simulink model "T6_changeloadmodeltocurrentload_v1"  (R2022b)
settings: Solver=FixedStepAuto  StartTime=0.0  StopTime=48*4  FixedStep=0.01  RelTol=1e-3
undefined symbols (not defined in the file): cableLV, cableMV, High, Low, LV, MV, Scaling_factor, Ts
libraries: fl_lib x149, nesl_utility x73, simulink x60, ee_lib x9
(part 2 of 3)

== system T6_changeloadmodeltocurrentload_v1/Household2 ==
  note: I = P / U
  Constant : Constant  Value=LV
  Controlled Current Source : fl_lib/Electrical/Electrical Sources/Controlled Current Source
  Current Sensor : fl_lib/Electrical/Electrical Sensors/Current Sensor
  Divide : Product  Inputs=*/
  Gain : Gain  Gain=Scaling_factor
  MATLAB Function : MATLAB Function  TreatAsAtomicUnit=on
  PS-Simulink Converter : nesl_utility/PS-Simulink Converter  PhysicalDomain=network_engine_domain  SubClassName=ps_output  LeftPortType=input  RightPortType=output  PseudoPeriodic=off  Frequencies=[]  VectorFormat=inherit  Unit=inherit  AffineConversion=off
  PS-Simulink Converter1 : nesl_utility/PS-Simulink Converter  PhysicalDomain=network_engine_domain  SubClassName=ps_output  LeftPortType=input  RightPortType=output  PseudoPeriodic=off  Frequencies=[]  VectorFormat=inherit  Unit=inherit  AffineConversion=off
  Product : Product
  Repeating Sequence Interpolated : simulink/Sources/Repeating Sequence Interpolated  OutValues=Household15_Springallday  TimeValues=Allday_timevector  LookUpMeth=Interpolation-Use End Values  tsamp=0.01  OutMin=[]  OutMax=[]  OutDataTypeStr=double  OutputDataTypeScalingMode=double  OutDataType=fixdt(0,8)  OutScaling=2^-10
  Repeating Sequence Interpolated1 : simulink/Sources/Repeating Sequence Interpolated  OutValues=Household15_Summerallday  TimeValues=Allday_timevector  LookUpMeth=Interpolation-Use End Values  tsamp=0.01  OutMin=[]  OutMax=[]  OutDataTypeStr=double  OutputDataTypeScalingMode=double  OutDataType=fixdt(0,8)  OutScaling=2^-10
  Repeating Sequence Interpolated2 : simulink/Sources/Repeating Sequence Interpolated  OutValues=Household15_Autumnallday  TimeValues=Allday_timevector  LookUpMeth=Interpolation-Use End Values  tsamp=0.01  OutMin=[]  OutMax=[]  OutDataTypeStr=double  OutputDataTypeScalingMode=double  OutDataType=fixdt(0,8)  OutScaling=2^-10
  Repeating Sequence Interpolated3 : simulink/Sources/Repeating Sequence Interpolated  OutValues=Household15_Winterallday  TimeValues=Allday_timevector  LookUpMeth=Interpolation-Use End Values  tsamp=0.01  OutMin=[]  OutMax=[]  OutDataTypeStr=double  OutputDataTypeScalingMode=double  OutDataType=fixdt(0,8)  OutScaling=2^-10
  Scope : Scope
  Simscape Bus1 : SimscapeBus  HierarchyStrings=High;Low
  Simulink-PS Converter1 : nesl_utility/Simulink-PS Converter  PhysicalDomain=network_engine_domain  SubClassName=ps_input  LeftPortType=input  RightPortType=output  PseudoPeriodic=off  Frequencies=[]  NoiseDistribution=none  NoiseParameters=[]  Unit=A  AffineConversion=off  FilteringAndDerivatives=provide  SimscapeFilterOrder=1  InputFilterTimeConstant=0.001  UdotUserProvided=0
  Voltage Sensor : fl_lib/Electrical/Electrical Sensors/Voltage Sensor
  IndustrialOut : PMIOPort  Side=Right
  tag scope: Residential_power2=global
  wires:
  Repeating Sequence Interpolated3/1 -> MATLAB Function/8(data4)
  Repeating Sequence Interpolated2/1 -> MATLAB Function/7(data3)
  Repeating Sequence Interpolated1/1 -> MATLAB Function/6(data2)
  Repeating Sequence Interpolated/1 -> MATLAB Function/5(data1)
  [Button1selected] -> MATLAB Function/1(button1)
  [Button2selected] -> MATLAB Function/2(button2)
  [Button3selected] -> MATLAB Function/3(button3)
  [Button4selected] -> MATLAB Function/4(button4)
  Product/1 -> [Residential_power2]  "power"
  PS-Simulink Converter1/1 -> Product/1  "current"
  PS-Simulink Converter/1 -> Product/2  "voltage"
  MATLAB Function/1(y) -> Gain/1, Scope/1  "electrical"
  Divide/1 -> Simulink-PS Converter1/1
  Gain/1 -> Divide/1
  Constant/1 -> Divide/2
  connections:
  Current Sensor/LConn1 -- Simscape Bus1/LConn1
  Current Sensor/RConn1 -- PS-Simulink Converter1/LConn1
  Voltage Sensor/RConn1 -- PS-Simulink Converter/LConn1
  Current Sensor/RConn2 -- Controlled Current Source/RConn2 -- Voltage Sensor/LConn1
  IndustrialOut/RConn1 -- Simscape Bus1/RConn1
  Voltage Sensor/RConn2 -- Simscape Bus1/LConn2 -- Controlled Current Source/LConn1
  Simulink-PS Converter1/RConn1 -- Controlled Current Source/RConn1

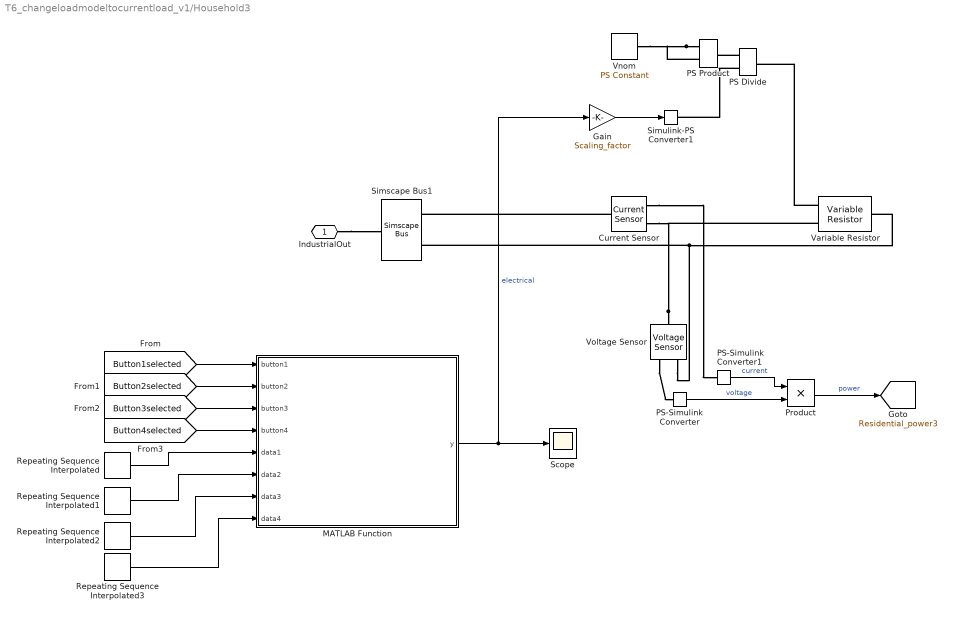
== system T6_changeloadmodeltocurrentload_v1/Household3 ==
  Current Sensor : fl_lib/Electrical/Electrical Sensors/Current Sensor
  Gain : Gain  Gain=Scaling_factor
  MATLAB Function : MATLAB Function  TreatAsAtomicUnit=on
  PS Divide : fl_lib/Physical Signals/Functions/PS Divide
  PS Product : fl_lib/Physical Signals/Functions/PS Product
  PS-Simulink Converter : nesl_utility/PS-Simulink Converter  PhysicalDomain=network_engine_domain  SubClassName=ps_output  LeftPortType=input  RightPortType=output  PseudoPeriodic=off  Frequencies=[]  VectorFormat=inherit  Unit=inherit  AffineConversion=off
  PS-Simulink Converter1 : nesl_utility/PS-Simulink Converter  PhysicalDomain=network_engine_domain  SubClassName=ps_output  LeftPortType=input  RightPortType=output  PseudoPeriodic=off  Frequencies=[]  VectorFormat=inherit  Unit=inherit  AffineConversion=off
  Product : Product
  Repeating Sequence Interpolated : simulink/Sources/Repeating Sequence Interpolated  OutValues=Household8_Springallday  TimeValues=Allday_timevector  LookUpMeth=Interpolation-Use End Values  tsamp=0.01  OutMin=[]  OutMax=[]  OutDataTypeStr=double  OutputDataTypeScalingMode=double  OutDataType=fixdt(0,8)  OutScaling=2^-10
  Repeating Sequence Interpolated1 : simulink/Sources/Repeating Sequence Interpolated  OutValues=Household8_Summerallday  TimeValues=Allday_timevector  LookUpMeth=Interpolation-Use End Values  tsamp=0.01  OutMin=[]  OutMax=[]  OutDataTypeStr=double  OutputDataTypeScalingMode=double  OutDataType=fixdt(0,8)  OutScaling=2^-10
  Repeating Sequence Interpolated2 : simulink/Sources/Repeating Sequence Interpolated  OutValues=Household8_Autumnallday  TimeValues=Allday_timevector  LookUpMeth=Interpolation-Use End Values  tsamp=0.01  OutMin=[]  OutMax=[]  OutDataTypeStr=double  OutputDataTypeScalingMode=double  OutDataType=fixdt(0,8)  OutScaling=2^-10
  Repeating Sequence Interpolated3 : simulink/Sources/Repeating Sequence Interpolated  OutValues=Household8_Winterallday  TimeValues=Allday_timevector  LookUpMeth=Interpolation-Use End Values  tsamp=0.01  OutMin=[]  OutMax=[]  OutDataTypeStr=double  OutputDataTypeScalingMode=double  OutDataType=fixdt(0,8)  OutScaling=2^-10
  Scope : Scope
  Simscape Bus1 : SimscapeBus  HierarchyStrings=High;Low
  Simulink-PS Converter1 : nesl_utility/Simulink-PS Converter  PhysicalDomain=network_engine_domain  SubClassName=ps_input  LeftPortType=input  RightPortType=output  PseudoPeriodic=off  Frequencies=[]  NoiseDistribution=none  NoiseParameters=[]  Unit=V*A  AffineConversion=off  FilteringAndDerivatives=provide  SimscapeFilterOrder=1  InputFilterTimeConstant=0.001  UdotUserProvided=0
  Variable Resistor : fl_lib/Electrical/Electrical Elements/Variable Resistor  Rmin=0 Ohm  i_specify=off  i_priority=None  i=0 A  i_nominal_specify=off  i_nominal_unit=A  i_nominal_value=1  v_specify=off  v_priority=None  v=0 V  v_nominal_specify=off  v_nominal_unit=V  v_nominal_value=1
  Vnom : fl_lib/Physical Signals/Sources/PS Constant  constant=LV V
  Voltage Sensor : fl_lib/Electrical/Electrical Sensors/Voltage Sensor
  IndustrialOut : PMIOPort  Side=Right
  tag scope: Residential_power3=global
  wires:
  MATLAB Function/1(y) -> Gain/1, Scope/1  "electrical"
  PS-Simulink Converter/1 -> Product/2  "voltage"
  PS-Simulink Converter1/1 -> Product/1  "current"
  Product/1 -> [Residential_power3]  "power"
  [Button4selected] -> MATLAB Function/4(button4)
  [Button3selected] -> MATLAB Function/3(button3)
  [Button2selected] -> MATLAB Function/2(button2)
  [Button1selected] -> MATLAB Function/1(button1)
  Repeating Sequence Interpolated/1 -> MATLAB Function/5(data1)
  Repeating Sequence Interpolated1/1 -> MATLAB Function/6(data2)
  Repeating Sequence Interpolated2/1 -> MATLAB Function/7(data3)
  Repeating Sequence Interpolated3/1 -> MATLAB Function/8(data4)
  Gain/1 -> Simulink-PS Converter1/1
  connections:
  PS Divide/LConn1 -- PS Product/RConn1
  Variable Resistor/LConn1 -- PS Divide/RConn1
  PS Divide/LConn2 -- Simulink-PS Converter1/RConn1
  PS Product/LConn1 -- PS Product/LConn2 -- Vnom/RConn1
  Voltage Sensor/RConn2 -- Simscape Bus1/LConn2 -- Variable Resistor/RConn1
  IndustrialOut/RConn1 -- Simscape Bus1/RConn1
  Voltage Sensor/LConn1 -- Variable Resistor/LConn2 -- Current Sensor/RConn2
  Voltage Sensor/RConn1 -- PS-Simulink Converter/LConn1
  Current Sensor/RConn1 -- PS-Simulink Converter1/LConn1
  Current Sensor/LConn1 -- Simscape Bus1/LConn1

== system T6_changeloadmodeltocurrentload_v1/Household4 ==
  Current Sensor : fl_lib/Electrical/Electrical Sensors/Current Sensor
  Gain : Gain  Gain=Scaling_factor
  MATLAB Function : MATLAB Function  TreatAsAtomicUnit=on
  PS Divide : fl_lib/Physical Signals/Functions/PS Divide
  PS Product : fl_lib/Physical Signals/Functions/PS Product
  PS-Simulink Converter : nesl_utility/PS-Simulink Converter  PhysicalDomain=network_engine_domain  SubClassName=ps_output  LeftPortType=input  RightPortType=output  PseudoPeriodic=off  Frequencies=[]  VectorFormat=inherit  Unit=inherit  AffineConversion=off
  PS-Simulink Converter1 : nesl_utility/PS-Simulink Converter  PhysicalDomain=network_engine_domain  SubClassName=ps_output  LeftPortType=input  RightPortType=output  PseudoPeriodic=off  Frequencies=[]  VectorFormat=inherit  Unit=inherit  AffineConversion=off
  Product : Product
  Repeating Sequence Interpolated : simulink/Sources/Repeating Sequence Interpolated  OutValues=Household4_Springallday  TimeValues=Allday_timevector  LookUpMeth=Interpolation-Use End Values  tsamp=0.01  OutMin=[]  OutMax=[]  OutDataTypeStr=double  OutputDataTypeScalingMode=double  OutDataType=fixdt(0,8)  OutScaling=2^-10
  Repeating Sequence Interpolated1 : simulink/Sources/Repeating Sequence Interpolated  OutValues=Household4_Summerallday  TimeValues=Allday_timevector  LookUpMeth=Interpolation-Use End Values  tsamp=0.01  OutMin=[]  OutMax=[]  OutDataTypeStr=double  OutputDataTypeScalingMode=double  OutDataType=fixdt(0,8)  OutScaling=2^-10
  Repeating Sequence Interpolated2 : simulink/Sources/Repeating Sequence Interpolated  OutValues=Household4_Autumnallday  TimeValues=Allday_timevector  LookUpMeth=Interpolation-Use End Values  tsamp=0.01  OutMin=[]  OutMax=[]  OutDataTypeStr=double  OutputDataTypeScalingMode=double  OutDataType=fixdt(0,8)  OutScaling=2^-10
  Repeating Sequence Interpolated3 : simulink/Sources/Repeating Sequence Interpolated  OutValues=Household4_Winterallday  TimeValues=Allday_timevector  LookUpMeth=Interpolation-Use End Values  tsamp=0.01  OutMin=[]  OutMax=[]  OutDataTypeStr=double  OutputDataTypeScalingMode=double  OutDataType=fixdt(0,8)  OutScaling=2^-10
  Scope : Scope
  Simscape Bus1 : SimscapeBus  HierarchyStrings=High;Low
  Simulink-PS Converter1 : nesl_utility/Simulink-PS Converter  PhysicalDomain=network_engine_domain  SubClassName=ps_input  LeftPortType=input  RightPortType=output  PseudoPeriodic=off  Frequencies=[]  NoiseDistribution=none  NoiseParameters=[]  Unit=V*A  AffineConversion=off  FilteringAndDerivatives=provide  SimscapeFilterOrder=1  InputFilterTimeConstant=0.001  UdotUserProvided=0
  Variable Resistor : fl_lib/Electrical/Electrical Elements/Variable Resistor  Rmin=0 Ohm  i_specify=off  i_priority=None  i=0 A  i_nominal_specify=off  i_nominal_unit=A  i_nominal_value=1  v_specify=off  v_priority=None  v=0 V  v_nominal_specify=off  v_nominal_unit=V  v_nominal_value=1
  Vnom : fl_lib/Physical Signals/Sources/PS Constant  constant=LV V
  Voltage Sensor : fl_lib/Electrical/Electrical Sensors/Voltage Sensor
  IndustrialOut : PMIOPort  Side=Right
  tag scope: Residential_power4=global
  wires:
  Repeating Sequence Interpolated3/1 -> MATLAB Function/8(data4)
  Repeating Sequence Interpolated2/1 -> MATLAB Function/7(data3)
  Repeating Sequence Interpolated1/1 -> MATLAB Function/6(data2)
  Repeating Sequence Interpolated/1 -> MATLAB Function/5(data1)
  [Button1selected] -> MATLAB Function/1(button1)
  [Button2selected] -> MATLAB Function/2(button2)
  [Button3selected] -> MATLAB Function/3(button3)
  [Button4selected] -> MATLAB Function/4(button4)
  Product/1 -> [Residential_power4]  "power"
  PS-Simulink Converter1/1 -> Product/1  "current"
  PS-Simulink Converter/1 -> Product/2  "voltage"
  MATLAB Function/1(y) -> Gain/1, Scope/1  "electrical"
  Gain/1 -> Simulink-PS Converter1/1
  connections:
  Current Sensor/LConn1 -- Simscape Bus1/LConn1
  Current Sensor/RConn1 -- PS-Simulink Converter1/LConn1
  Voltage Sensor/RConn1 -- PS-Simulink Converter/LConn1
  Current Sensor/RConn2 -- Variable Resistor/LConn2 -- Voltage Sensor/LConn1
  IndustrialOut/RConn1 -- Simscape Bus1/RConn1
  Variable Resistor/RConn1 -- Simscape Bus1/LConn2 -- Voltage Sensor/RConn2
  Vnom/RConn1 -- PS Product/LConn2 -- PS Product/LConn1
  PS Divide/LConn2 -- Simulink-PS Converter1/RConn1
  Variable Resistor/LConn1 -- PS Divide/RConn1
  PS Divide/LConn1 -- PS Product/RConn1

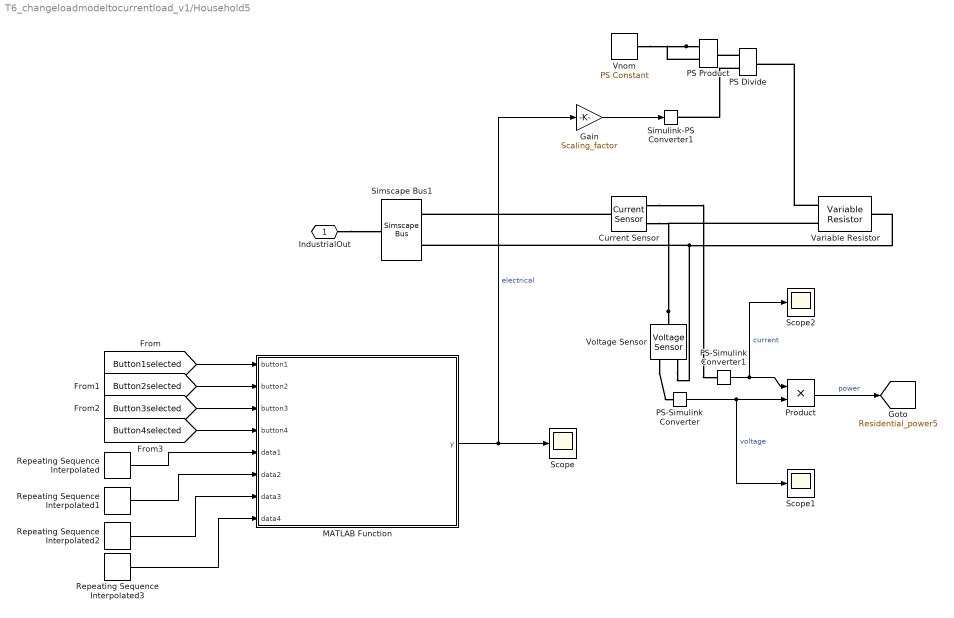
== system T6_changeloadmodeltocurrentload_v1/Household5 ==
  Current Sensor : fl_lib/Electrical/Electrical Sensors/Current Sensor
  Gain : Gain  Gain=Scaling_factor
  MATLAB Function : MATLAB Function  TreatAsAtomicUnit=on
  PS Divide : fl_lib/Physical Signals/Functions/PS Divide
  PS Product : fl_lib/Physical Signals/Functions/PS Product
  PS-Simulink Converter : nesl_utility/PS-Simulink Converter  PhysicalDomain=network_engine_domain  SubClassName=ps_output  LeftPortType=input  RightPortType=output  PseudoPeriodic=off  Frequencies=[]  VectorFormat=inherit  Unit=inherit  AffineConversion=off
  PS-Simulink Converter1 : nesl_utility/PS-Simulink Converter  PhysicalDomain=network_engine_domain  SubClassName=ps_output  LeftPortType=input  RightPortType=output  PseudoPeriodic=off  Frequencies=[]  VectorFormat=inherit  Unit=inherit  AffineConversion=off
  Product : Product
  Repeating Sequence Interpolated : simulink/Sources/Repeating Sequence Interpolated  OutValues=Household26_Springallday  TimeValues=Allday_timevector  LookUpMeth=Interpolation-Use End Values  tsamp=0.01  OutMin=[]  OutMax=[]  OutDataTypeStr=double  OutputDataTypeScalingMode=double  OutDataType=fixdt(0,8)  OutScaling=2^-10
  Repeating Sequence Interpolated1 : simulink/Sources/Repeating Sequence Interpolated  OutValues=Household26_Summerallday  TimeValues=Allday_timevector  LookUpMeth=Interpolation-Use End Values  tsamp=0.01  OutMin=[]  OutMax=[]  OutDataTypeStr=double  OutputDataTypeScalingMode=double  OutDataType=fixdt(0,8)  OutScaling=2^-10
  Repeating Sequence Interpolated2 : simulink/Sources/Repeating Sequence Interpolated  OutValues=Household26_Autumnallday  TimeValues=Allday_timevector  LookUpMeth=Interpolation-Use End Values  tsamp=0.01  OutMin=[]  OutMax=[]  OutDataTypeStr=double  OutputDataTypeScalingMode=double  OutDataType=fixdt(0,8)  OutScaling=2^-10
  Repeating Sequence Interpolated3 : simulink/Sources/Repeating Sequence Interpolated  OutValues=Household26_Winterallday  TimeValues=Allday_timevector  LookUpMeth=Interpolation-Use End Values  tsamp=0.01  OutMin=[]  OutMax=[]  OutDataTypeStr=double  OutputDataTypeScalingMode=double  OutDataType=fixdt(0,8)  OutScaling=2^-10
  Scope : Scope
  Scope1 : Scope
  Scope2 : Scope
  Simscape Bus1 : SimscapeBus  HierarchyStrings=High;Low
  Simulink-PS Converter1 : nesl_utility/Simulink-PS Converter  PhysicalDomain=network_engine_domain  SubClassName=ps_input  LeftPortType=input  RightPortType=output  PseudoPeriodic=off  Frequencies=[]  NoiseDistribution=none  NoiseParameters=[]  Unit=V*A  AffineConversion=off  FilteringAndDerivatives=provide  SimscapeFilterOrder=1  InputFilterTimeConstant=0.001  UdotUserProvided=0
  Variable Resistor : fl_lib/Electrical/Electrical Elements/Variable Resistor  Rmin=0 Ohm  i_specify=off  i_priority=None  i=0 A  i_nominal_specify=off  i_nominal_unit=A  i_nominal_value=1  v_specify=off  v_priority=None  v=0 V  v_nominal_specify=off  v_nominal_unit=V  v_nominal_value=1
  Vnom : fl_lib/Physical Signals/Sources/PS Constant  constant=LV V
  Voltage Sensor : fl_lib/Electrical/Electrical Sensors/Voltage Sensor
  IndustrialOut : PMIOPort  Side=Right
  tag scope: Residential_power5=global
  wires:
  MATLAB Function/1(y) -> Gain/1, Scope/1  "electrical"
  PS-Simulink Converter/1 -> Scope1/1, Product/2  "voltage"
  PS-Simulink Converter1/1 -> Scope2/1, Product/1  "current"
  Product/1 -> [Residential_power5]  "power"
  [Button4selected] -> MATLAB Function/4(button4)
  [Button3selected] -> MATLAB Function/3(button3)
  [Button2selected] -> MATLAB Function/2(button2)
  [Button1selected] -> MATLAB Function/1(button1)
  Repeating Sequence Interpolated/1 -> MATLAB Function/5(data1)
  Repeating Sequence Interpolated1/1 -> MATLAB Function/6(data2)
  Repeating Sequence Interpolated2/1 -> MATLAB Function/7(data3)
  Repeating Sequence Interpolated3/1 -> MATLAB Function/8(data4)
  Gain/1 -> Simulink-PS Converter1/1
  connections:
  PS Divide/LConn1 -- PS Product/RConn1
  Variable Resistor/LConn1 -- PS Divide/RConn1
  PS Divide/LConn2 -- Simulink-PS Converter1/RConn1
  PS Product/LConn1 -- PS Product/LConn2 -- Vnom/RConn1
  Voltage Sensor/RConn2 -- Simscape Bus1/LConn2 -- Variable Resistor/RConn1
  IndustrialOut/RConn1 -- Simscape Bus1/RConn1
  Voltage Sensor/LConn1 -- Variable Resistor/LConn2 -- Current Sensor/RConn2
  Voltage Sensor/RConn1 -- PS-Simulink Converter/LConn1
  Current Sensor/RConn1 -- PS-Simulink Converter1/LConn1
  Current Sensor/LConn1 -- Simscape Bus1/LConn1

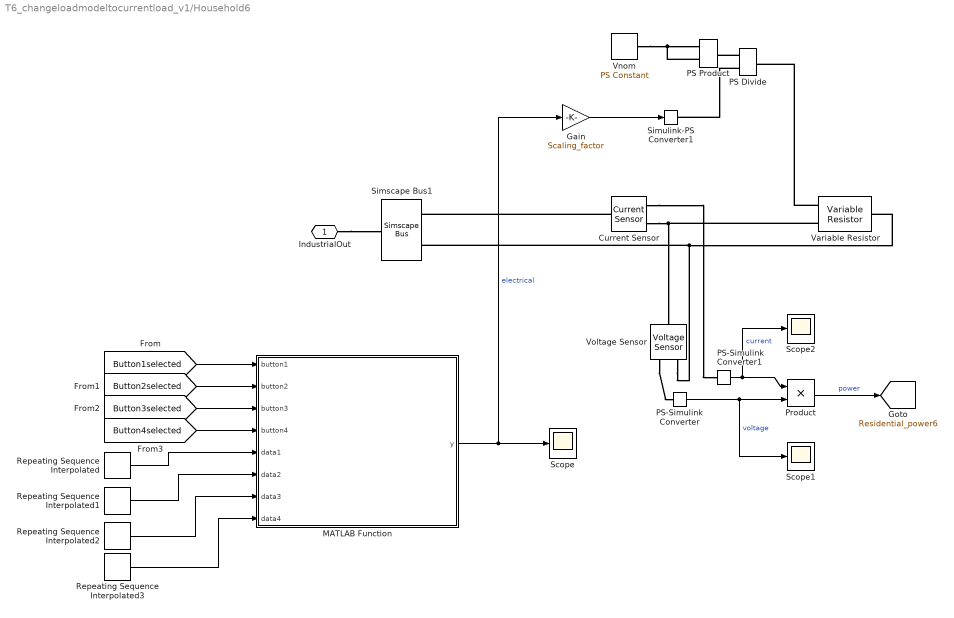
== system T6_changeloadmodeltocurrentload_v1/Household6 ==
  Current Sensor : fl_lib/Electrical/Electrical Sensors/Current Sensor
  Gain : Gain  Gain=Scaling_factor
  MATLAB Function : MATLAB Function  TreatAsAtomicUnit=on
  PS Divide : fl_lib/Physical Signals/Functions/PS Divide
  PS Product : fl_lib/Physical Signals/Functions/PS Product
  PS-Simulink Converter : nesl_utility/PS-Simulink Converter  PhysicalDomain=network_engine_domain  SubClassName=ps_output  LeftPortType=input  RightPortType=output  PseudoPeriodic=off  Frequencies=[]  VectorFormat=inherit  Unit=inherit  AffineConversion=off
  PS-Simulink Converter1 : nesl_utility/PS-Simulink Converter  PhysicalDomain=network_engine_domain  SubClassName=ps_output  LeftPortType=input  RightPortType=output  PseudoPeriodic=off  Frequencies=[]  VectorFormat=inherit  Unit=inherit  AffineConversion=off
  Product : Product
  Repeating Sequence Interpolated : simulink/Sources/Repeating Sequence Interpolated  OutValues=Household9_Springallday  TimeValues=Allday_timevector  LookUpMeth=Interpolation-Use End Values  tsamp=0.01  OutMin=[]  OutMax=[]  OutDataTypeStr=double  OutputDataTypeScalingMode=double  OutDataType=fixdt(0,8)  OutScaling=2^-10
  Repeating Sequence Interpolated1 : simulink/Sources/Repeating Sequence Interpolated  OutValues=Household9_Summerallday  TimeValues=Allday_timevector  LookUpMeth=Interpolation-Use End Values  tsamp=0.01  OutMin=[]  OutMax=[]  OutDataTypeStr=double  OutputDataTypeScalingMode=double  OutDataType=fixdt(0,8)  OutScaling=2^-10
  Repeating Sequence Interpolated2 : simulink/Sources/Repeating Sequence Interpolated  OutValues=Household9_Autumnallday  TimeValues=Allday_timevector  LookUpMeth=Interpolation-Use End Values  tsamp=0.01  OutMin=[]  OutMax=[]  OutDataTypeStr=double  OutputDataTypeScalingMode=double  OutDataType=fixdt(0,8)  OutScaling=2^-10
  Repeating Sequence Interpolated3 : simulink/Sources/Repeating Sequence Interpolated  OutValues=Household9_Winterallday  TimeValues=Allday_timevector  LookUpMeth=Interpolation-Use End Values  tsamp=0.01  OutMin=[]  OutMax=[]  OutDataTypeStr=double  OutputDataTypeScalingMode=double  OutDataType=fixdt(0,8)  OutScaling=2^-10
  Scope : Scope
  Scope1 : Scope
  Scope2 : Scope
  Simscape Bus1 : SimscapeBus  HierarchyStrings=High;Low
  Simulink-PS Converter1 : nesl_utility/Simulink-PS Converter  PhysicalDomain=network_engine_domain  SubClassName=ps_input  LeftPortType=input  RightPortType=output  PseudoPeriodic=off  Frequencies=[]  NoiseDistribution=none  NoiseParameters=[]  Unit=V*A  AffineConversion=off  FilteringAndDerivatives=provide  SimscapeFilterOrder=1  InputFilterTimeConstant=0.001  UdotUserProvided=0
  Variable Resistor : fl_lib/Electrical/Electrical Elements/Variable Resistor  Rmin=0 Ohm  i_specify=off  i_priority=None  i=0 A  i_nominal_specify=off  i_nominal_unit=A  i_nominal_value=1  v_specify=off  v_priority=None  v=0 V  v_nominal_specify=off  v_nominal_unit=V  v_nominal_value=1
  Vnom : fl_lib/Physical Signals/Sources/PS Constant  constant=LV V
  Voltage Sensor : fl_lib/Electrical/Electrical Sensors/Voltage Sensor
  IndustrialOut : PMIOPort  Side=Right
  tag scope: Residential_power6=global
  wires:
  Repeating Sequence Interpolated3/1 -> MATLAB Function/8(data4)
  Repeating Sequence Interpolated2/1 -> MATLAB Function/7(data3)
  Repeating Sequence Interpolated1/1 -> MATLAB Function/6(data2)
  Repeating Sequence Interpolated/1 -> MATLAB Function/5(data1)
  [Button1selected] -> MATLAB Function/1(button1)
  [Button2selected] -> MATLAB Function/2(button2)
  [Button3selected] -> MATLAB Function/3(button3)
  [Button4selected] -> MATLAB Function/4(button4)
  Product/1 -> [Residential_power6]  "power"
  PS-Simulink Converter1/1 -> Scope2/1, Product/1  "current"
  PS-Simulink Converter/1 -> Scope1/1, Product/2  "voltage"
  MATLAB Function/1(y) -> Gain/1, Scope/1  "electrical"
  Gain/1 -> Simulink-PS Converter1/1
  connections:
  Current Sensor/LConn1 -- Simscape Bus1/LConn1
  Current Sensor/RConn1 -- PS-Simulink Converter1/LConn1
  Voltage Sensor/RConn1 -- PS-Simulink Converter/LConn1
  Current Sensor/RConn2 -- Variable Resistor/LConn2 -- Voltage Sensor/LConn1
  IndustrialOut/RConn1 -- Simscape Bus1/RConn1
  Variable Resistor/RConn1 -- Simscape Bus1/LConn2 -- Voltage Sensor/RConn2
  Vnom/RConn1 -- PS Product/LConn2 -- PS Product/LConn1
  PS Divide/LConn2 -- Simulink-PS Converter1/RConn1
  Variable Resistor/LConn1 -- PS Divide/RConn1
  PS Divide/LConn1 -- PS Product/RConn1

== system T6_changeloadmodeltocurrentload_v1/Household7 ==
  Current Sensor : fl_lib/Electrical/Electrical Sensors/Current Sensor
  Gain : Gain  Gain=Scaling_factor
  MATLAB Function : MATLAB Function  TreatAsAtomicUnit=on
  PS Divide : fl_lib/Physical Signals/Functions/PS Divide
  PS Product : fl_lib/Physical Signals/Functions/PS Product
  PS-Simulink Converter : nesl_utility/PS-Simulink Converter  PhysicalDomain=network_engine_domain  SubClassName=ps_output  LeftPortType=input  RightPortType=output  PseudoPeriodic=off  Frequencies=[]  VectorFormat=inherit  Unit=inherit  AffineConversion=off
  PS-Simulink Converter1 : nesl_utility/PS-Simulink Converter  PhysicalDomain=network_engine_domain  SubClassName=ps_output  LeftPortType=input  RightPortType=output  PseudoPeriodic=off  Frequencies=[]  VectorFormat=inherit  Unit=inherit  AffineConversion=off
  Product : Product
  Repeating Sequence Interpolated : simulink/Sources/Repeating Sequence Interpolated  OutValues=Household5_Springallday  TimeValues=Allday_timevector  LookUpMeth=Interpolation-Use End Values  tsamp=0.01  OutMin=[]  OutMax=[]  OutDataTypeStr=double  OutputDataTypeScalingMode=double  OutDataType=fixdt(0,8)  OutScaling=2^-10
  Repeating Sequence Interpolated1 : simulink/Sources/Repeating Sequence Interpolated  OutValues=Household5_Summerallday  TimeValues=Allday_timevector  LookUpMeth=Interpolation-Use End Values  tsamp=0.01  OutMin=[]  OutMax=[]  OutDataTypeStr=double  OutputDataTypeScalingMode=double  OutDataType=fixdt(0,8)  OutScaling=2^-10
  Repeating Sequence Interpolated2 : simulink/Sources/Repeating Sequence Interpolated  OutValues=Household5_Autumnallday  TimeValues=Allday_timevector  LookUpMeth=Interpolation-Use End Values  tsamp=0.01  OutMin=[]  OutMax=[]  OutDataTypeStr=double  OutputDataTypeScalingMode=double  OutDataType=fixdt(0,8)  OutScaling=2^-10
  Repeating Sequence Interpolated3 : simulink/Sources/Repeating Sequence Interpolated  OutValues=Household5_Winterallday  TimeValues=Allday_timevector  LookUpMeth=Interpolation-Use End Values  tsamp=0.01  OutMin=[]  OutMax=[]  OutDataTypeStr=double  OutputDataTypeScalingMode=double  OutDataType=fixdt(0,8)  OutScaling=2^-10
  Scope : Scope
  Simscape Bus1 : SimscapeBus  HierarchyStrings=High;Low
  Simulink-PS Converter1 : nesl_utility/Simulink-PS Converter  PhysicalDomain=network_engine_domain  SubClassName=ps_input  LeftPortType=input  RightPortType=output  PseudoPeriodic=off  Frequencies=[]  NoiseDistribution=none  NoiseParameters=[]  Unit=V*A  AffineConversion=off  FilteringAndDerivatives=provide  SimscapeFilterOrder=1  InputFilterTimeConstant=0.001  UdotUserProvided=0
  Variable Resistor : fl_lib/Electrical/Electrical Elements/Variable Resistor  Rmin=0 Ohm  i_specify=off  i_priority=None  i=0 A  i_nominal_specify=off  i_nominal_unit=A  i_nominal_value=1  v_specify=off  v_priority=None  v=0 V  v_nominal_specify=off  v_nominal_unit=V  v_nominal_value=1
  Vnom : fl_lib/Physical Signals/Sources/PS Constant  constant=LV V
  Voltage Sensor : fl_lib/Electrical/Electrical Sensors/Voltage Sensor
  IndustrialOut : PMIOPort  Side=Right
  tag scope: Residential_power7=global
  wires:
  MATLAB Function/1(y) -> Gain/1, Scope/1  "electrical"
  PS-Simulink Converter/1 -> Product/2  "voltage"
  PS-Simulink Converter1/1 -> Product/1  "current"
  Product/1 -> [Residential_power7]  "power"
  [Button4selected] -> MATLAB Function/4(button4)
  [Button3selected] -> MATLAB Function/3(button3)
  [Button2selected] -> MATLAB Function/2(button2)
  [Button1selected] -> MATLAB Function/1(button1)
  Repeating Sequence Interpolated/1 -> MATLAB Function/5(data1)
  Repeating Sequence Interpolated1/1 -> MATLAB Function/6(data2)
  Repeating Sequence Interpolated2/1 -> MATLAB Function/7(data3)
  Repeating Sequence Interpolated3/1 -> MATLAB Function/8(data4)
  Gain/1 -> Simulink-PS Converter1/1
  connections:
  PS Divide/LConn1 -- PS Product/RConn1
  Variable Resistor/LConn1 -- PS Divide/RConn1
  PS Divide/LConn2 -- Simulink-PS Converter1/RConn1
  PS Product/LConn1 -- PS Product/LConn2 -- Vnom/RConn1
  Voltage Sensor/RConn2 -- Simscape Bus1/LConn2 -- Variable Resistor/RConn1
  IndustrialOut/RConn1 -- Simscape Bus1/RConn1
  Voltage Sensor/LConn1 -- Variable Resistor/LConn2 -- Current Sensor/RConn2
  Voltage Sensor/RConn1 -- PS-Simulink Converter/LConn1
  Current Sensor/RConn1 -- PS-Simulink Converter1/LConn1
  Current Sensor/LConn1 -- Simscape Bus1/LConn1

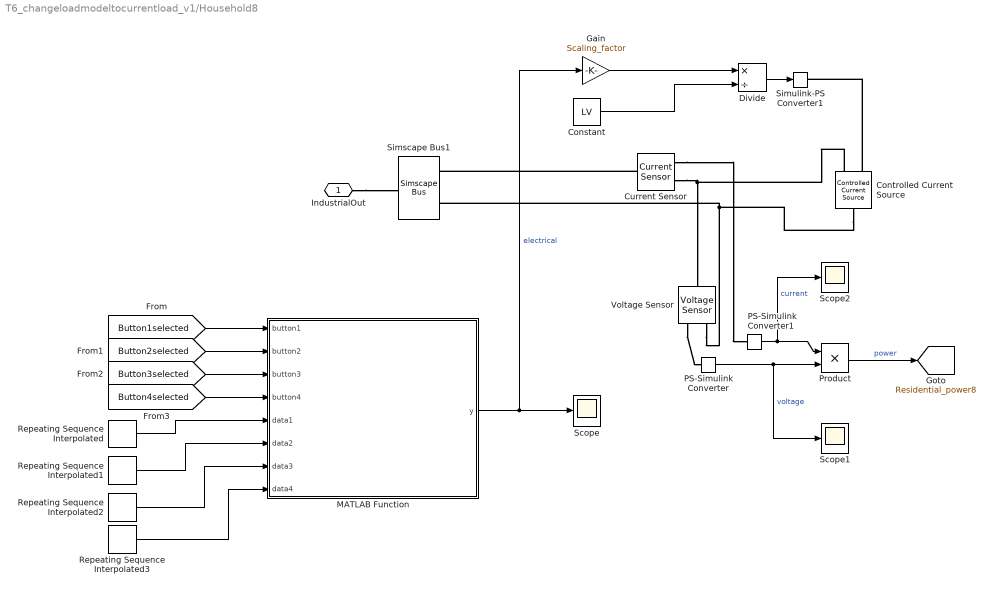
== system T6_changeloadmodeltocurrentload_v1/Household8 ==
  Constant : Constant  Value=LV
  Controlled Current Source : fl_lib/Electrical/Electrical Sources/Controlled Current Source
  Current Sensor : fl_lib/Electrical/Electrical Sensors/Current Sensor
  Divide : Product  Inputs=*/
  Gain : Gain  Gain=Scaling_factor
  MATLAB Function : MATLAB Function  TreatAsAtomicUnit=on
  PS-Simulink Converter : nesl_utility/PS-Simulink Converter  PhysicalDomain=network_engine_domain  SubClassName=ps_output  LeftPortType=input  RightPortType=output  PseudoPeriodic=off  Frequencies=[]  VectorFormat=inherit  Unit=inherit  AffineConversion=off
  PS-Simulink Converter1 : nesl_utility/PS-Simulink Converter  PhysicalDomain=network_engine_domain  SubClassName=ps_output  LeftPortType=input  RightPortType=output  PseudoPeriodic=off  Frequencies=[]  VectorFormat=inherit  Unit=inherit  AffineConversion=off
  Product : Product
  Repeating Sequence Interpolated : simulink/Sources/Repeating Sequence Interpolated  OutValues=Household33_Springallday  TimeValues=Allday_timevector  LookUpMeth=Interpolation-Use End Values  tsamp=0.01  OutMin=[]  OutMax=[]  OutDataTypeStr=double  OutputDataTypeScalingMode=double  OutDataType=fixdt(0,8)  OutScaling=2^-10
  Repeating Sequence Interpolated1 : simulink/Sources/Repeating Sequence Interpolated  OutValues=Household33_Summerallday  TimeValues=Allday_timevector  LookUpMeth=Interpolation-Use End Values  tsamp=0.01  OutMin=[]  OutMax=[]  OutDataTypeStr=double  OutputDataTypeScalingMode=double  OutDataType=fixdt(0,8)  OutScaling=2^-10
  Repeating Sequence Interpolated2 : simulink/Sources/Repeating Sequence Interpolated  OutValues=Household33_Autumnallday  TimeValues=Allday_timevector  LookUpMeth=Interpolation-Use End Values  tsamp=0.01  OutMin=[]  OutMax=[]  OutDataTypeStr=double  OutputDataTypeScalingMode=double  OutDataType=fixdt(0,8)  OutScaling=2^-10
  Repeating Sequence Interpolated3 : simulink/Sources/Repeating Sequence Interpolated  OutValues=Household33_Winterallday  TimeValues=Allday_timevector  LookUpMeth=Interpolation-Use End Values  tsamp=0.01  OutMin=[]  OutMax=[]  OutDataTypeStr=double  OutputDataTypeScalingMode=double  OutDataType=fixdt(0,8)  OutScaling=2^-10
  Scope : Scope
  Scope1 : Scope
  Scope2 : Scope
  Simscape Bus1 : SimscapeBus  HierarchyStrings=High;Low
  Simulink-PS Converter1 : nesl_utility/Simulink-PS Converter  PhysicalDomain=network_engine_domain  SubClassName=ps_input  LeftPortType=input  RightPortType=output  PseudoPeriodic=off  Frequencies=[]  NoiseDistribution=none  NoiseParameters=[]  Unit=A  AffineConversion=off  FilteringAndDerivatives=provide  SimscapeFilterOrder=1  InputFilterTimeConstant=0.001  UdotUserProvided=0
  Voltage Sensor : fl_lib/Electrical/Electrical Sensors/Voltage Sensor
  IndustrialOut : PMIOPort  Side=Right
  tag scope: Residential_power8=global
  wires:
  Repeating Sequence Interpolated3/1 -> MATLAB Function/8(data4)
  Repeating Sequence Interpolated2/1 -> MATLAB Function/7(data3)
  Repeating Sequence Interpolated1/1 -> MATLAB Function/6(data2)
  Repeating Sequence Interpolated/1 -> MATLAB Function/5(data1)
  [Button1selected] -> MATLAB Function/1(button1)
  [Button2selected] -> MATLAB Function/2(button2)
  [Button3selected] -> MATLAB Function/3(button3)
  [Button4selected] -> MATLAB Function/4(button4)
  Product/1 -> [Residential_power8]  "power"
  PS-Simulink Converter1/1 -> Scope2/1, Product/1  "current"
  PS-Simulink Converter/1 -> Scope1/1, Product/2  "voltage"
  MATLAB Function/1(y) -> Gain/1, Scope/1  "electrical"
  Divide/1 -> Simulink-PS Converter1/1
  Gain/1 -> Divide/1
  Constant/1 -> Divide/2
  connections:
  Current Sensor/LConn1 -- Simscape Bus1/LConn1
  Current Sensor/RConn1 -- PS-Simulink Converter1/LConn1
  Voltage Sensor/RConn1 -- PS-Simulink Converter/LConn1
  Current Sensor/RConn2 -- Controlled Current Source/RConn2 -- Voltage Sensor/LConn1
  IndustrialOut/RConn1 -- Simscape Bus1/RConn1
  Voltage Sensor/RConn2 -- Controlled Current Source/LConn1 -- Simscape Bus1/LConn2
  Controlled Current Source/RConn1 -- Simulink-PS Converter1/RConn1

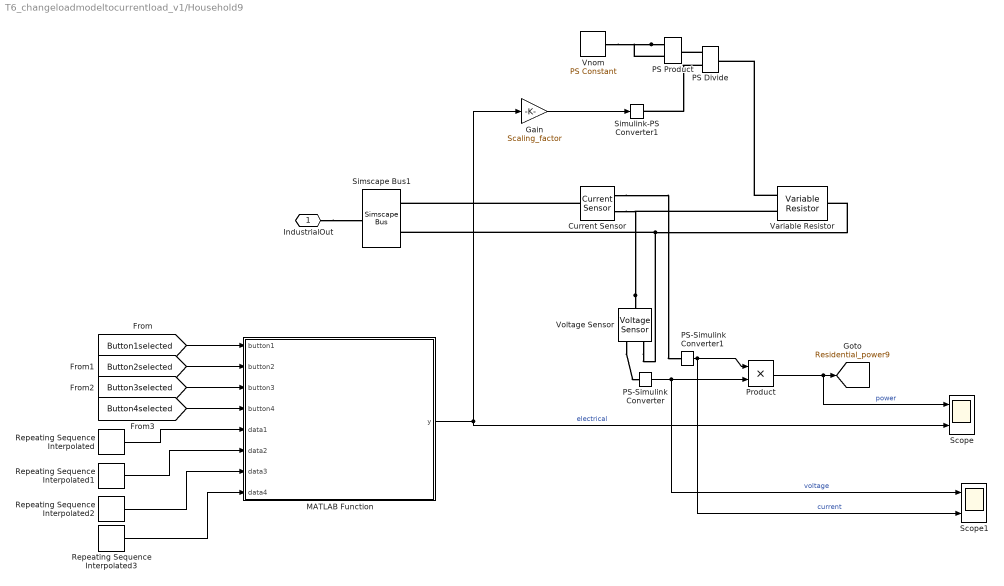
== system T6_changeloadmodeltocurrentload_v1/Household9 ==
  Current Sensor : fl_lib/Electrical/Electrical Sensors/Current Sensor
  Gain : Gain  Gain=Scaling_factor
  MATLAB Function : MATLAB Function  TreatAsAtomicUnit=on
  PS Divide : fl_lib/Physical Signals/Functions/PS Divide
  PS Product : fl_lib/Physical Signals/Functions/PS Product
  PS-Simulink Converter : nesl_utility/PS-Simulink Converter  PhysicalDomain=network_engine_domain  SubClassName=ps_output  LeftPortType=input  RightPortType=output  PseudoPeriodic=off  Frequencies=[]  VectorFormat=inherit  Unit=inherit  AffineConversion=off
  PS-Simulink Converter1 : nesl_utility/PS-Simulink Converter  PhysicalDomain=network_engine_domain  SubClassName=ps_output  LeftPortType=input  RightPortType=output  PseudoPeriodic=off  Frequencies=[]  VectorFormat=inherit  Unit=inherit  AffineConversion=off
  Product : Product
  Repeating Sequence Interpolated : simulink/Sources/Repeating Sequence Interpolated  OutValues=Household10_Springallday  TimeValues=Allday_timevector  LookUpMeth=Interpolation-Use End Values  tsamp=0.01  OutMin=[]  OutMax=[]  OutDataTypeStr=double  OutputDataTypeScalingMode=double  OutDataType=fixdt(0,8)  OutScaling=2^-10
  Repeating Sequence Interpolated1 : simulink/Sources/Repeating Sequence Interpolated  OutValues=Household10_Summerallday  TimeValues=Allday_timevector  LookUpMeth=Interpolation-Use End Values  tsamp=0.01  OutMin=[]  OutMax=[]  OutDataTypeStr=double  OutputDataTypeScalingMode=double  OutDataType=fixdt(0,8)  OutScaling=2^-10
  Repeating Sequence Interpolated2 : simulink/Sources/Repeating Sequence Interpolated  OutValues=Household10_Autumnallday  TimeValues=Allday_timevector  LookUpMeth=Interpolation-Use End Values  tsamp=0.01  OutMin=[]  OutMax=[]  OutDataTypeStr=double  OutputDataTypeScalingMode=double  OutDataType=fixdt(0,8)  OutScaling=2^-10
  Repeating Sequence Interpolated3 : simulink/Sources/Repeating Sequence Interpolated  OutValues=Household10_Winterallday  TimeValues=Allday_timevector  LookUpMeth=Interpolation-Use End Values  tsamp=0.01  OutMin=[]  OutMax=[]  OutDataTypeStr=double  OutputDataTypeScalingMode=double  OutDataType=fixdt(0,8)  OutScaling=2^-10
  Scope : Scope  NumInputPorts=2
  Scope1 : Scope  NumInputPorts=2
  Simscape Bus1 : SimscapeBus  HierarchyStrings=High;Low
  Simulink-PS Converter1 : nesl_utility/Simulink-PS Converter  PhysicalDomain=network_engine_domain  SubClassName=ps_input  LeftPortType=input  RightPortType=output  PseudoPeriodic=off  Frequencies=[]  NoiseDistribution=none  NoiseParameters=[]  Unit=V*A  AffineConversion=off  FilteringAndDerivatives=provide  SimscapeFilterOrder=1  InputFilterTimeConstant=0.001  UdotUserProvided=0
  Variable Resistor : fl_lib/Electrical/Electrical Elements/Variable Resistor  Rmin=0 Ohm  i_specify=off  i_priority=None  i=0 A  i_nominal_specify=off  i_nominal_unit=A  i_nominal_value=1  v_specify=off  v_priority=None  v=0 V  v_nominal_specify=off  v_nominal_unit=V  v_nominal_value=1
  Vnom : fl_lib/Physical Signals/Sources/PS Constant  constant=LV V
  Voltage Sensor : fl_lib/Electrical/Electrical Sensors/Voltage Sensor
  IndustrialOut : PMIOPort  Side=Right
  tag scope: Residential_power9=global
  wires:
  MATLAB Function/1(y) -> Scope/2, Gain/1  "electrical"
  PS-Simulink Converter/1 -> Scope1/1, Product/2  "voltage"
  PS-Simulink Converter1/1 -> Scope1/2, Product/1  "current"
  Product/1 -> Scope/1, [Residential_power9]  "power"
  [Button4selected] -> MATLAB Function/4(button4)
  [Button3selected] -> MATLAB Function/3(button3)
  [Button2selected] -> MATLAB Function/2(button2)
  [Button1selected] -> MATLAB Function/1(button1)
  Repeating Sequence Interpolated/1 -> MATLAB Function/5(data1)
  Repeating Sequence Interpolated1/1 -> MATLAB Function/6(data2)
  Repeating Sequence Interpolated2/1 -> MATLAB Function/7(data3)
  Repeating Sequence Interpolated3/1 -> MATLAB Function/8(data4)
  Gain/1 -> Simulink-PS Converter1/1
  connections:
  PS Divide/LConn1 -- PS Product/RConn1
  Variable Resistor/LConn1 -- PS Divide/RConn1
  PS Divide/LConn2 -- Simulink-PS Converter1/RConn1
  PS Product/LConn1 -- PS Product/LConn2 -- Vnom/RConn1
  Voltage Sensor/RConn2 -- Simscape Bus1/LConn2 -- Variable Resistor/RConn1
  IndustrialOut/RConn1 -- Simscape Bus1/RConn1
  Voltage Sensor/LConn1 -- Variable Resistor/LConn2 -- Current Sensor/RConn2
  Voltage Sensor/RConn1 -- PS-Simulink Converter/LConn1
  Current Sensor/RConn1 -- PS-Simulink Converter1/LConn1
  Current Sensor/LConn1 -- Simscape Bus1/LConn1

== system T6_changeloadmodeltocurrentload_v1/Line1 ==
  Resistor : fl_lib/Electrical/Electrical Elements/Resistor  R=rho*l/A Ohm  i_specify=off  i_priority=None  i=0 A  i_nominal_specify=off  i_nominal_unit=A  i_nominal_value=1  v_specify=off  v_priority=None  v=0 V  v_nominal_specify=off  v_nominal_unit=V  v_nominal_value=1
  Resistor1 : fl_lib/Electrical/Electrical Elements/Resistor  R=rho*l/A Ohm  i_specify=off  i_priority=None  i=0 A  i_nominal_specify=off  i_nominal_unit=A  i_nominal_value=1  v_specify=off  v_priority=None  v=0 V  v_nominal_specify=off  v_nominal_unit=V  v_nominal_value=1
  Simscape Bus2 : SimscapeBus  HierarchyStrings=High;Low
  Simscape Bus3 : SimscapeBus  HierarchyStrings=High;Low
  In : PMIOPort  Side=Left
  Out : PMIOPort  Port=2  Side=Right
  connections:
  Simscape Bus2/LConn1 -- Resistor/LConn1
  Simscape Bus3/LConn2 -- Resistor1/RConn1
  Simscape Bus2/RConn1 -- In/RConn1
  Simscape Bus3/LConn1 -- Resistor/RConn1
  Resistor1/LConn1 -- Simscape Bus2/LConn2
  Simscape Bus3/RConn1 -- Out/RConn1

== system T6_changeloadmodeltocurrentload_v1/Line10 ==
  Resistor : fl_lib/Electrical/Electrical Elements/Resistor  R=rho*l/A Ohm  i_specify=off  i_priority=None  i=0 A  i_nominal_specify=off  i_nominal_unit=A  i_nominal_value=1  v_specify=off  v_priority=None  v=0 V  v_nominal_specify=off  v_nominal_unit=V  v_nominal_value=1
  Resistor1 : fl_lib/Electrical/Electrical Elements/Resistor  R=rho*l/A Ohm  i_specify=off  i_priority=None  i=0 A  i_nominal_specify=off  i_nominal_unit=A  i_nominal_value=1  v_specify=off  v_priority=None  v=0 V  v_nominal_specify=off  v_nominal_unit=V  v_nominal_value=1
  Simscape Bus2 : SimscapeBus  HierarchyStrings=High;Low
  Simscape Bus3 : SimscapeBus  HierarchyStrings=High;Low
  In : PMIOPort  Side=Left
  Out : PMIOPort  Port=2  Side=Right
  connections:
  Simscape Bus2/LConn1 -- Resistor/LConn1
  Simscape Bus3/LConn2 -- Resistor1/RConn1
  Simscape Bus2/RConn1 -- In/RConn1
  Simscape Bus3/LConn1 -- Resistor/RConn1
  Resistor1/LConn1 -- Simscape Bus2/LConn2
  Simscape Bus3/RConn1 -- Out/RConn1

== system T6_changeloadmodeltocurrentload_v1/Line11 ==
  Resistor : fl_lib/Electrical/Electrical Elements/Resistor  R=rho*l/A Ohm  i_specify=off  i_priority=None  i=0 A  i_nominal_specify=off  i_nominal_unit=A  i_nominal_value=1  v_specify=off  v_priority=None  v=0 V  v_nominal_specify=off  v_nominal_unit=V  v_nominal_value=1
  Resistor1 : fl_lib/Electrical/Electrical Elements/Resistor  R=rho*l/A Ohm  i_specify=off  i_priority=None  i=0 A  i_nominal_specify=off  i_nominal_unit=A  i_nominal_value=1  v_specify=off  v_priority=None  v=0 V  v_nominal_specify=off  v_nominal_unit=V  v_nominal_value=1
  Simscape Bus2 : SimscapeBus  HierarchyStrings=High;Low
  Simscape Bus3 : SimscapeBus  HierarchyStrings=High;Low
  In : PMIOPort  Side=Left
  Out : PMIOPort  Port=2  Side=Right
  connections:
  Simscape Bus3/RConn1 -- Out/RConn1
  Resistor1/LConn1 -- Simscape Bus2/LConn2
  Simscape Bus3/LConn1 -- Resistor/RConn1
  Simscape Bus2/RConn1 -- In/RConn1
  Simscape Bus3/LConn2 -- Resistor1/RConn1
  Simscape Bus2/LConn1 -- Resistor/LConn1

== system T6_changeloadmodeltocurrentload_v1/Line12 ==
  Resistor : fl_lib/Electrical/Electrical Elements/Resistor  R=rho*l/A Ohm  i_specify=off  i_priority=None  i=0 A  i_nominal_specify=off  i_nominal_unit=A  i_nominal_value=1  v_specify=off  v_priority=None  v=0 V  v_nominal_specify=off  v_nominal_unit=V  v_nominal_value=1
  Resistor1 : fl_lib/Electrical/Electrical Elements/Resistor  R=rho*l/A Ohm  i_specify=off  i_priority=None  i=0 A  i_nominal_specify=off  i_nominal_unit=A  i_nominal_value=1  v_specify=off  v_priority=None  v=0 V  v_nominal_specify=off  v_nominal_unit=V  v_nominal_value=1
  Simscape Bus2 : SimscapeBus  HierarchyStrings=High;Low
  Simscape Bus3 : SimscapeBus  HierarchyStrings=High;Low
  In : PMIOPort  Side=Left
  Out : PMIOPort  Port=2  Side=Right
  connections:
  Simscape Bus3/RConn1 -- Out/RConn1
  Resistor1/LConn1 -- Simscape Bus2/LConn2
  Simscape Bus3/LConn1 -- Resistor/RConn1
  Simscape Bus2/RConn1 -- In/RConn1
  Simscape Bus3/LConn2 -- Resistor1/RConn1
  Simscape Bus2/LConn1 -- Resistor/LConn1

== system T6_changeloadmodeltocurrentload_v1/Line13 ==
  Resistor : fl_lib/Electrical/Electrical Elements/Resistor  R=rho*l/A Ohm  i_specify=off  i_priority=None  i=0 A  i_nominal_specify=off  i_nominal_unit=A  i_nominal_value=1  v_specify=off  v_priority=None  v=0 V  v_nominal_specify=off  v_nominal_unit=V  v_nominal_value=1
  Resistor1 : fl_lib/Electrical/Electrical Elements/Resistor  R=rho*l/A Ohm  i_specify=off  i_priority=None  i=0 A  i_nominal_specify=off  i_nominal_unit=A  i_nominal_value=1  v_specify=off  v_priority=None  v=0 V  v_nominal_specify=off  v_nominal_unit=V  v_nominal_value=1
  Simscape Bus2 : SimscapeBus  HierarchyStrings=High;Low
  Simscape Bus3 : SimscapeBus  HierarchyStrings=High;Low
  In : PMIOPort  Side=Left
  Out : PMIOPort  Port=2  Side=Right
  connections:
  Simscape Bus2/LConn1 -- Resistor/LConn1
  Simscape Bus3/LConn2 -- Resistor1/RConn1
  Simscape Bus2/RConn1 -- In/RConn1
  Simscape Bus3/LConn1 -- Resistor/RConn1
  Resistor1/LConn1 -- Simscape Bus2/LConn2
  Simscape Bus3/RConn1 -- Out/RConn1

== system T6_changeloadmodeltocurrentload_v1/Line14 ==
  Resistor : fl_lib/Electrical/Electrical Elements/Resistor  R=rho*l/A Ohm  i_specify=off  i_priority=None  i=0 A  i_nominal_specify=off  i_nominal_unit=A  i_nominal_value=1  v_specify=off  v_priority=None  v=0 V  v_nominal_specify=off  v_nominal_unit=V  v_nominal_value=1
  Resistor1 : fl_lib/Electrical/Electrical Elements/Resistor  R=rho*l/A Ohm  i_specify=off  i_priority=None  i=0 A  i_nominal_specify=off  i_nominal_unit=A  i_nominal_value=1  v_specify=off  v_priority=None  v=0 V  v_nominal_specify=off  v_nominal_unit=V  v_nominal_value=1
  Simscape Bus2 : SimscapeBus  HierarchyStrings=High;Low
  Simscape Bus3 : SimscapeBus  HierarchyStrings=High;Low
  In : PMIOPort  Side=Left
  Out : PMIOPort  Port=2  Side=Right
  connections:
  Simscape Bus3/RConn1 -- Out/RConn1
  Resistor1/LConn1 -- Simscape Bus2/LConn2
  Simscape Bus3/LConn1 -- Resistor/RConn1
  Simscape Bus2/RConn1 -- In/RConn1
  Simscape Bus3/LConn2 -- Resistor1/RConn1
  Simscape Bus2/LConn1 -- Resistor/LConn1

== system T6_changeloadmodeltocurrentload_v1/Line15 ==
  Resistor : fl_lib/Electrical/Electrical Elements/Resistor  R=rho*l/A Ohm  i_specify=off  i_priority=None  i=0 A  i_nominal_specify=off  i_nominal_unit=A  i_nominal_value=1  v_specify=off  v_priority=None  v=0 V  v_nominal_specify=off  v_nominal_unit=V  v_nominal_value=1
  Resistor1 : fl_lib/Electrical/Electrical Elements/Resistor  R=rho*l/A Ohm  i_specify=off  i_priority=None  i=0 A  i_nominal_specify=off  i_nominal_unit=A  i_nominal_value=1  v_specify=off  v_priority=None  v=0 V  v_nominal_specify=off  v_nominal_unit=V  v_nominal_value=1
  Simscape Bus2 : SimscapeBus  HierarchyStrings=High;Low
  Simscape Bus3 : SimscapeBus  HierarchyStrings=High;Low
  In : PMIOPort  Side=Left
  Out : PMIOPort  Port=2  Side=Right
  connections:
  Simscape Bus2/LConn1 -- Resistor/LConn1
  Simscape Bus3/LConn2 -- Resistor1/RConn1
  Simscape Bus2/RConn1 -- In/RConn1
  Simscape Bus3/LConn1 -- Resistor/RConn1
  Resistor1/LConn1 -- Simscape Bus2/LConn2
  Simscape Bus3/RConn1 -- Out/RConn1

== system T6_changeloadmodeltocurrentload_v1/Line16 ==
  Resistor : fl_lib/Electrical/Electrical Elements/Resistor  R=rho*l/A Ohm  i_specify=off  i_priority=None  i=0 A  i_nominal_specify=off  i_nominal_unit=A  i_nominal_value=1  v_specify=off  v_priority=None  v=0 V  v_nominal_specify=off  v_nominal_unit=V  v_nominal_value=1
  Resistor1 : fl_lib/Electrical/Electrical Elements/Resistor  R=rho*l/A Ohm  i_specify=off  i_priority=None  i=0 A  i_nominal_specify=off  i_nominal_unit=A  i_nominal_value=1  v_specify=off  v_priority=None  v=0 V  v_nominal_specify=off  v_nominal_unit=V  v_nominal_value=1
  Simscape Bus2 : SimscapeBus  HierarchyStrings=High;Low
  Simscape Bus3 : SimscapeBus  HierarchyStrings=High;Low
  In : PMIOPort  Side=Left
  Out : PMIOPort  Port=2  Side=Right
  connections:
  Simscape Bus2/LConn1 -- Resistor/LConn1
  Simscape Bus3/LConn2 -- Resistor1/RConn1
  Simscape Bus2/RConn1 -- In/RConn1
  Simscape Bus3/LConn1 -- Resistor/RConn1
  Resistor1/LConn1 -- Simscape Bus2/LConn2
  Simscape Bus3/RConn1 -- Out/RConn1

== system T6_changeloadmodeltocurrentload_v1/Line17 ==
  Resistor : fl_lib/Electrical/Electrical Elements/Resistor  R=rho*l/A Ohm  i_specify=off  i_priority=None  i=0 A  i_nominal_specify=off  i_nominal_unit=A  i_nominal_value=1  v_specify=off  v_priority=None  v=0 V  v_nominal_specify=off  v_nominal_unit=V  v_nominal_value=1
  Resistor1 : fl_lib/Electrical/Electrical Elements/Resistor  R=rho*l/A Ohm  i_specify=off  i_priority=None  i=0 A  i_nominal_specify=off  i_nominal_unit=A  i_nominal_value=1  v_specify=off  v_priority=None  v=0 V  v_nominal_specify=off  v_nominal_unit=V  v_nominal_value=1
  Simscape Bus2 : SimscapeBus  HierarchyStrings=High;Low
  Simscape Bus3 : SimscapeBus  HierarchyStrings=High;Low
  In : PMIOPort  Side=Left
  Out : PMIOPort  Port=2  Side=Right
  connections:
  Simscape Bus3/RConn1 -- Out/RConn1
  Resistor1/LConn1 -- Simscape Bus2/LConn2
  Simscape Bus3/LConn1 -- Resistor/RConn1
  Simscape Bus2/RConn1 -- In/RConn1
  Simscape Bus3/LConn2 -- Resistor1/RConn1
  Simscape Bus2/LConn1 -- Resistor/LConn1

== system T6_changeloadmodeltocurrentload_v1/Line18 ==
  Resistor : fl_lib/Electrical/Electrical Elements/Resistor  R=rho*l/A Ohm  i_specify=off  i_priority=None  i=0 A  i_nominal_specify=off  i_nominal_unit=A  i_nominal_value=1  v_specify=off  v_priority=None  v=0 V  v_nominal_specify=off  v_nominal_unit=V  v_nominal_value=1
  Resistor1 : fl_lib/Electrical/Electrical Elements/Resistor  R=rho*l/A Ohm  i_specify=off  i_priority=None  i=0 A  i_nominal_specify=off  i_nominal_unit=A  i_nominal_value=1  v_specify=off  v_priority=None  v=0 V  v_nominal_specify=off  v_nominal_unit=V  v_nominal_value=1
  Simscape Bus2 : SimscapeBus  HierarchyStrings=High;Low
  Simscape Bus3 : SimscapeBus  HierarchyStrings=High;Low
  In : PMIOPort  Side=Left
  Out : PMIOPort  Port=2  Side=Right
  connections:
  Simscape Bus3/RConn1 -- Out/RConn1
  Resistor1/LConn1 -- Simscape Bus2/LConn2
  Simscape Bus3/LConn1 -- Resistor/RConn1
  Simscape Bus2/RConn1 -- In/RConn1
  Simscape Bus3/LConn2 -- Resistor1/RConn1
  Simscape Bus2/LConn1 -- Resistor/LConn1

== system T6_changeloadmodeltocurrentload_v1/Line19 ==
  Current Sensor : fl_lib/Electrical/Electrical Sensors/Current Sensor
  PS-Simulink Converter : nesl_utility/PS-Simulink Converter  PhysicalDomain=network_engine_domain  SubClassName=ps_output  LeftPortType=input  RightPortType=output  PseudoPeriodic=off  Frequencies=[]  VectorFormat=inherit  Unit=inherit  AffineConversion=off
  Resistor : fl_lib/Electrical/Electrical Elements/Resistor  R=rho*l/A Ohm  i_specify=off  i_priority=None  i=0 A  i_nominal_specify=off  i_nominal_unit=A  i_nominal_value=1  v_specify=off  v_priority=None  v=0 V  v_nominal_specify=off  v_nominal_unit=V  v_nominal_value=1
  Resistor1 : fl_lib/Electrical/Electrical Elements/Resistor  R=rho*l/A Ohm  i_specify=off  i_priority=None  i=0 A  i_nominal_specify=off  i_nominal_unit=A  i_nominal_value=1  v_specify=off  v_priority=None  v=0 V  v_nominal_specify=off  v_nominal_unit=V  v_nominal_value=1
  Scope : Scope
  Simscape Bus2 : SimscapeBus  HierarchyStrings=High;Low
  Simscape Bus3 : SimscapeBus  HierarchyStrings=High;Low
  In : PMIOPort  Side=Left
  Out : PMIOPort  Port=2  Side=Right
  wires:
  PS-Simulink Converter/1 -> Scope/1
  connections:
  Simscape Bus2/LConn1 -- Resistor/LConn1
  Simscape Bus3/LConn2 -- Resistor1/RConn1
  Simscape Bus2/RConn1 -- In/RConn1
  Resistor1/LConn1 -- Simscape Bus2/LConn2
  Simscape Bus3/RConn1 -- Out/RConn1
  PS-Simulink Converter/LConn1 -- Current Sensor/RConn1
  Resistor/RConn1 -- Current Sensor/LConn1
  Current Sensor/RConn2 -- Simscape Bus3/LConn1

== system T6_changeloadmodeltocurrentload_v1/Line2 ==
  Resistor : fl_lib/Electrical/Electrical Elements/Resistor  R=rho*l/A Ohm  i_specify=off  i_priority=None  i=0 A  i_nominal_specify=off  i_nominal_unit=A  i_nominal_value=1  v_specify=off  v_priority=None  v=0 V  v_nominal_specify=off  v_nominal_unit=V  v_nominal_value=1
  Resistor1 : fl_lib/Electrical/Electrical Elements/Resistor  R=rho*l/A Ohm  i_specify=off  i_priority=None  i=0 A  i_nominal_specify=off  i_nominal_unit=A  i_nominal_value=1  v_specify=off  v_priority=None  v=0 V  v_nominal_specify=off  v_nominal_unit=V  v_nominal_value=1
  Simscape Bus2 : SimscapeBus  HierarchyStrings=High;Low
  Simscape Bus3 : SimscapeBus  HierarchyStrings=High;Low
  In : PMIOPort  Side=Left
  Out : PMIOPort  Port=2  Side=Right
  connections:
  Simscape Bus3/RConn1 -- Out/RConn1
  Resistor1/LConn1 -- Simscape Bus2/LConn2
  Simscape Bus3/LConn1 -- Resistor/RConn1
  Simscape Bus2/RConn1 -- In/RConn1
  Simscape Bus3/LConn2 -- Resistor1/RConn1
  Simscape Bus2/LConn1 -- Resistor/LConn1

== system T6_changeloadmodeltocurrentload_v1/Line20 ==
  Resistor : fl_lib/Electrical/Electrical Elements/Resistor  R=rho*l/A Ohm  i_specify=off  i_priority=None  i=0 A  i_nominal_specify=off  i_nominal_unit=A  i_nominal_value=1  v_specify=off  v_priority=None  v=0 V  v_nominal_specify=off  v_nominal_unit=V  v_nominal_value=1
  Resistor1 : fl_lib/Electrical/Electrical Elements/Resistor  R=rho*l/A Ohm  i_specify=off  i_priority=None  i=0 A  i_nominal_specify=off  i_nominal_unit=A  i_nominal_value=1  v_specify=off  v_priority=None  v=0 V  v_nominal_specify=off  v_nominal_unit=V  v_nominal_value=1
  Simscape Bus2 : SimscapeBus  HierarchyStrings=High;Low
  Simscape Bus3 : SimscapeBus  HierarchyStrings=High;Low
  In : PMIOPort  Side=Left
  Out : PMIOPort  Port=2  Side=Right
  connections:
  Simscape Bus3/RConn1 -- Out/RConn1
  Resistor1/LConn1 -- Simscape Bus2/LConn2
  Simscape Bus3/LConn1 -- Resistor/RConn1
  Simscape Bus2/RConn1 -- In/RConn1
  Simscape Bus3/LConn2 -- Resistor1/RConn1
  Simscape Bus2/LConn1 -- Resistor/LConn1
